simulink model "vertical"  (R2025a)
settings: Solver=VariableStepAuto  StartTime=0.0  StopTime=10.0  RelTol=1e-3
settings Model: Creator=marce  LastModifiedBy=marce

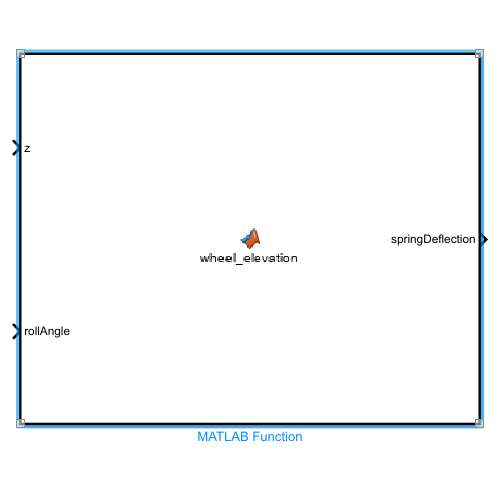
[thumbnail: Simulink's stored preview of the top-level diagram]
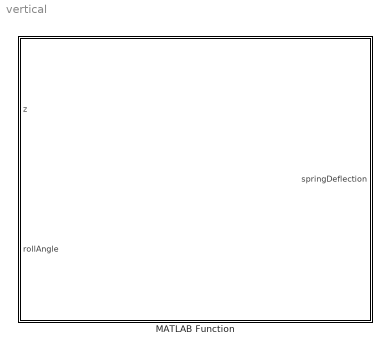
== system vertical ==
  MATLAB Function : MATLAB Function  TreatAsAtomicUnit=on

== matlab function vertical/MATLAB Function ==
  data: z input; rollAngle input; springDeflection output
function springDeflection  = wheel_elevation(z, rollAngle)
    
    springDeflection = z * ones(4,1) + sin(rollAngle) * [-0.5; 0.5; -0.5; 0.5] * [trackWidthF; trackWidthF; trackWidthR; trackWidthR]....
        + sin(pitchAngle) * [distancePitchCentreF; distancePitchCentreF; distancePitchCentreR; distancePitchCentreR];
